simulink model "DhwStationPId3d4"  (R2017a)
settings: Solver=FixedStepAuto  StartTime=-100  StopTime=100  FixedStep=dt  RelTol=1e-3
values from neighbouring files (symbols this model uses):
  A_0 = [ 0.7687, 0,      0,      0.1258, 0,      0,      12.31;          0.1054, 0.7687, 0,      0,      0.1258, 0,      12.31;          0,      0.1054, 0.7687, 0,      0,      0.1258, 12.31;          0.1161, 0,      0,      0.7867, 0.0972, 0,      0.7009;          0,      0.1161, 0,      0,      0.7867, 0.0972, 0.7009;          0,      0,      0.1161, 0,      0,      0.7867, 0.7009;          0,      0,  ...(+44 chars)    [LoadTruncatedSystemMatrices.m]
  A_1 = [	0,  0,  0,  0,  0,  0,  1.054;          0,  0,  0,  0,  0,  0,  0;          0,  0,  0,  0,  0,  0,  0;          0,  0,  0,  0,  0,  0,  0;          0,  0,  0,  0,  0,  0,  0;          0,  0,  0,  0,  0,  0,  0;          0,  0,  0,  0,  0,  0,  0]    [LoadTruncatedSystemMatrices.m]
  A_3 = 1e-3*[    -0.0597,0,      0,      0.0597,     0,  0,      0;                  0,      -0.0597,0,      0,      0.0597, 0,      0;                  0,      0,      -0.0597,0,      0,      0.0597, 0;                  0.0551, 0,      0 ,     -972.4, 972.4,  0,      0;                  0,      0.0551, 0,      0,      -972.4, 972.4,  0;                  0,      0, 0.0551,      0,      0,      -972.4, 0; ...(+68 chars)    [LoadTruncatedSystemMatrices.m]
  A_4 = [ -1.127, 0     , 0,      0.0731, 0,      0,          0;          1.054,  -1.127, 0,      0,      0.0731, 0,          0;          0,      1.054,  -1.127, 0,      0,      0.0731,     0;          0.0675, 0,      0,      -0.0675,0,      0,          0;          0,      0.0675, 0,      0,      -0.0675,0,          0;          0,      0,      0.0675, 0,      0,      -0.0675,    0;          0,      0,     ...(+40 chars)    [LoadTruncatedSystemMatrices.m]
  B_0 = [	0,	0,	0,	0,	0,	0, 0.1]'    [LoadTruncatedSystemMatrices.m]
  C = [0, 0, 0, 1, 0,  0,  0]    [LoadTruncatedSystemMatrices.m]
  d_0 = [70, 	10, 0.1, 0.1]    [LoadTruncatedSystemMatrices.m]
  dt = 0.1    [LoadTruncatedSystemMatrices.m]
  G_1 = [0.1054,	0,	0,	0,	0,	0,	0]'    [LoadTruncatedSystemMatrices.m]
  G_2 = [0, 0, 0,	0, 0, 0.0972, 0]'    [LoadTruncatedSystemMatrices.m]
  G_23 = [ 0,	0,	0,	0,	0, 0.9724,	0]'    [LoadTruncatedSystemMatrices.m]
  G_3 = [ -.0006,	-.0006,	-.0006,	-12.05,	-12.05,	-12.05, 0]'    [LoadTruncatedSystemMatrices.m]
  PId3d4_Ki = 0.000139128218356    [OptimizationReults_GainScheduledPId3d4.mat]    (also in OptimizeGainScheduledPId3d4.m = double(Ki))
  PId3d4_Kid3 = 0.000268812937216    [OptimizationReults_GainScheduledPId3d4.mat]    (also in OptimizeGainScheduledPId3d4.m = double(Kid3))
  PId3d4_Kid3d4 = -0.000522259839167    [OptimizationReults_GainScheduledPId3d4.mat]    (also in OptimizeGainScheduledPId3d4.m = double(Kid3d4))
  PId3d4_Kid4 = 0.000317478765518    [OptimizationReults_GainScheduledPId3d4.mat]    (also in OptimizeGainScheduledPId3d4.m = double(Kid4))
  PId3d4_Kp = 0.0070026798963    [OptimizationReults_GainScheduledPId3d4.mat]    (also in OptimizeGainScheduledPId3d4.m = double(Kp))
  PId3d4_Kpd3 = -0.00260700779742    [OptimizationReults_GainScheduledPId3d4.mat]    (also in OptimizeGainScheduledPId3d4.m = double(Kpd3))
  PId3d4_Kpd3d4 = -0.0177923584549    [OptimizationReults_GainScheduledPId3d4.mat]    (also in OptimizeGainScheduledPId3d4.m = double(Kpd3d4))
  PId3d4_Kpd4 = -0.00285749425693    [OptimizationReults_GainScheduledPId3d4.mat]    (also in OptimizeGainScheduledPId3d4.m = double(Kpd4))
  u_0 = 0.1    [LoadTruncatedSystemMatrices.m]
  x_0 = [ 57.5979, 45.1957, 32.7936,	47.2064, 34.8043, 22.4021, 0.1]'    [LoadTruncatedSystemMatrices.m]
  y_0 = C*x_0    [LoadTruncatedSystemMatrices.m]
settings Model: Creator=tgrunert  LastModifiedBy=tgrunert
settings OptimizationCC: DefaultParameterBehavior=Inlined

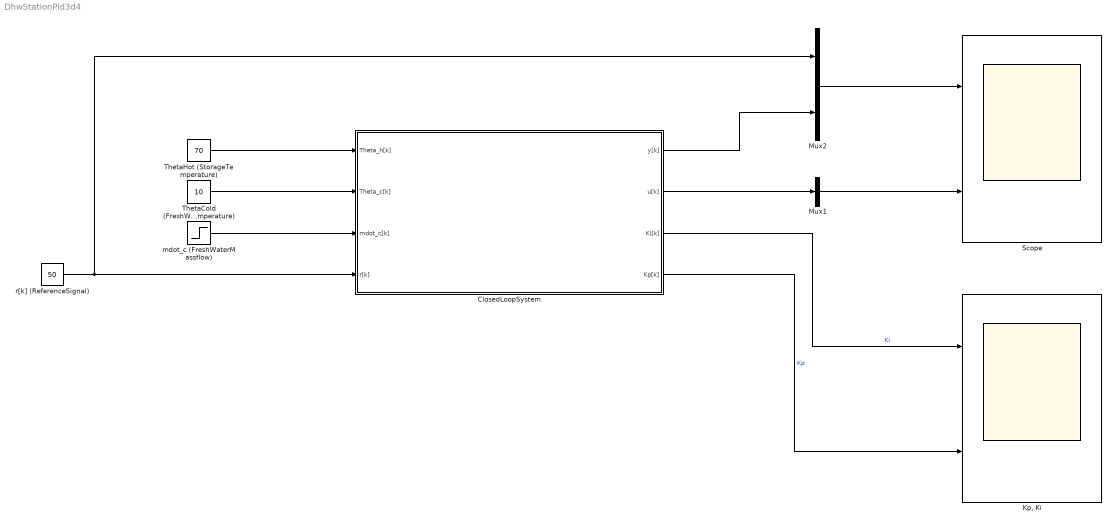
== system DhwStationPId3d4 ==
  ClosedLoopSystem : Subsystem
  "Kp, Ki" : Scope  NumInputPorts=2
  Mux1 : Mux  Inputs=1
  Mux2 : Mux  Inputs=2
  Scope : Scope  NumInputPorts=2
  ThetaCold (FreshWaterTemperature) : Constant  Value=10
  ThetaHot (StorageTemperature) : Constant  Value=70
  mdot_c (FreshWaterMassflow) : Step  Time=0  Before=0.125  After=0.075  SampleTime=0
  r[k] (ReferenceSignal) : Constant  Value=50
  wires:
  Mux1/1 -> Scope/2
  Mux2/1 -> Scope/1
  r[k] (ReferenceSignal)/1 -> Mux2/1, ClosedLoopSystem/4(r[k])
  ThetaCold (FreshWaterTemperature)/1 -> ClosedLoopSystem/2(Theta_c[k])
  ClosedLoopSystem/1(y[k]) -> Mux2/2
  ClosedLoopSystem/2(u[k]) -> Mux1/1
  ThetaHot (StorageTemperature)/1 -> ClosedLoopSystem/1(Theta_h[k])
  mdot_c (FreshWaterMassflow)/1 -> ClosedLoopSystem/3(mdot_c[k])
  ClosedLoopSystem/3(Ki[k]) -> "Kp, Ki"/1  "Ki"
  ClosedLoopSystem/4(Kp[k]) -> "Kp, Ki"/2  "Kp"

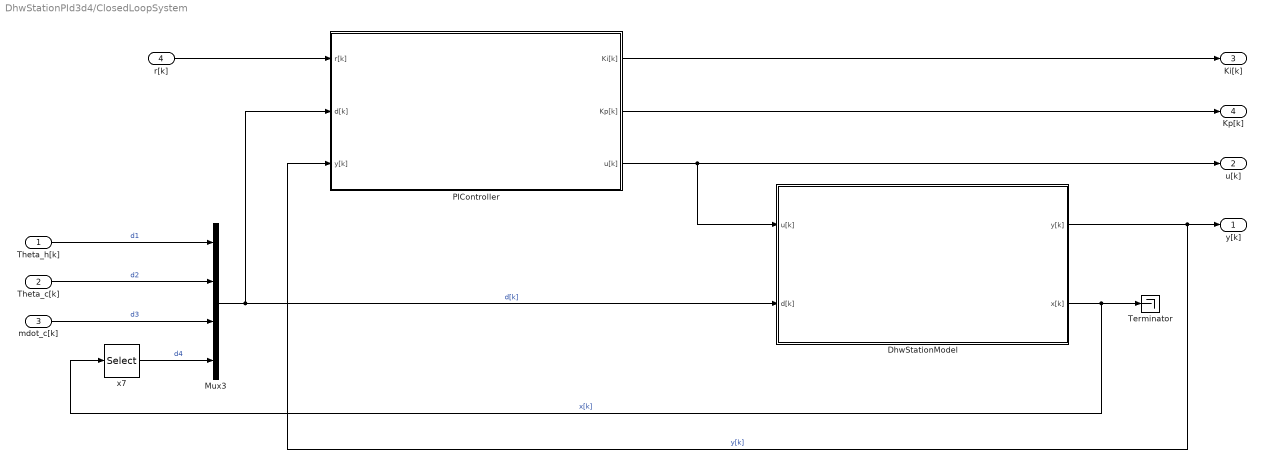
== system DhwStationPId3d4/ClosedLoopSystem ==
  Theta_h[k] : Inport
  Theta_c[k] : Inport  Port=2
  mdot_c[k] : Inport  Port=3
  r[k] : Inport  Port=4
  DhwStationModel : Subsystem  SystemSampleTime=dt
  Mux3 : Mux
  PIController : Subsystem
  Terminator : Terminator
  x7 : Selector  InputPortWidth=7  IndexOptions=Index vector (dialog)  Indices=[7]  OutputSizes=1
  y[k] : Outport
  u[k] : Outport  Port=2
  Ki[k] : Outport  Port=3
  Kp[k] : Outport  Port=4
  wires:
  PIController/3(u[k]) -> u[k]/1, DhwStationModel/1(u[k])
  DhwStationModel/2(x[k]) -> x7/1, Terminator/1  "x[k]"
  Theta_c[k]/1 -> Mux3/2  "d2"
  DhwStationModel/1(y[k]) -> y[k]/1, PIController/3(y[k])  "y[k]"
  Theta_h[k]/1 -> Mux3/1  "d1"
  mdot_c[k]/1 -> Mux3/3  "d3"
  Mux3/1 -> PIController/2(d[k]), DhwStationModel/2(d[k])  "d[k]"
  r[k]/1 -> PIController/1(r[k])
  x7/1 -> Mux3/4  "d4"
  PIController/1(Ki[k]) -> Ki[k]/1
  PIController/2(Kp[k]) -> Kp[k]/1

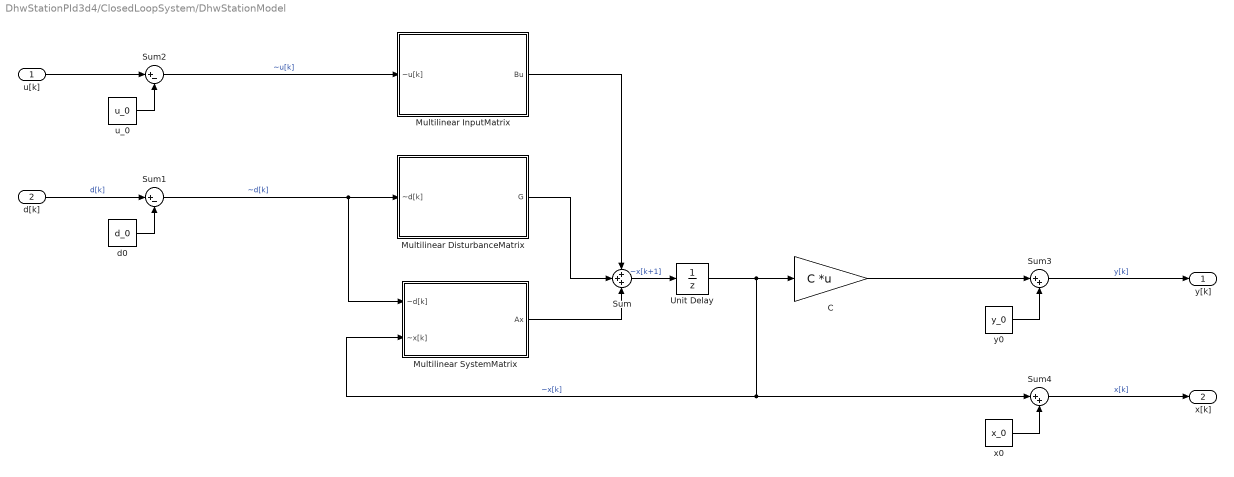
== system DhwStationPId3d4/ClosedLoopSystem/DhwStationModel ==
  u[k] : Inport
  d[k] : Inport  Port=2
  C : Gain  Gain=C  Multiplication=Matrix(K*u) (u vector)
  Multilinear DisturbanceMatrix : Subsystem
  Multilinear InputMatrix : Subsystem
  Multilinear SystemMatrix : Subsystem
  Sum : Sum  Inputs=+++
  Sum1 : Sum  Inputs=|+-
  Sum2 : Sum  Inputs=|+-
  Sum3 : Sum  Inputs=|++
  Sum4 : Sum  Inputs=|++
  Unit Delay : UnitDelay  SampleTime=-1
  d0 : Constant  Value=d_0
  u_0 : Constant  Value=u_0
  "x0 " : Constant  Value=x_0
  y0 : Constant  Value=y_0
  y[k] : Outport  PortDimensions=1
  x[k] : Outport  Port=2
  wires:
  Sum4/1 -> x[k]/1  "x[k]"
  "x0 "/1 -> Sum4/2
  y0/1 -> Sum3/2
  Sum3/1 -> y[k]/1  "y[k]"
  d0/1 -> Sum1/2
  d[k]/1 -> Sum1/1  "d[k]"
  C/1 -> Sum3/1
  Multilinear InputMatrix/1(Bu) -> Sum/1
  Multilinear SystemMatrix/1(Ax) -> Sum/3
  Unit Delay/1 -> Multilinear SystemMatrix/2(~x[k]), Sum4/1, C/1  "~x[k]"
  Sum/1 -> Unit Delay/1  "~x[k+1]"
  u[k]/1 -> Sum2/1
  u_0/1 -> Sum2/2
  Sum2/1 -> Multilinear InputMatrix/1(~u[k])  "~u[k]"
  Multilinear DisturbanceMatrix/1(G) -> Sum/2
  Sum1/1 -> Multilinear SystemMatrix/1(~d[k]), Multilinear DisturbanceMatrix/1(~d[k])  "~d[k]"

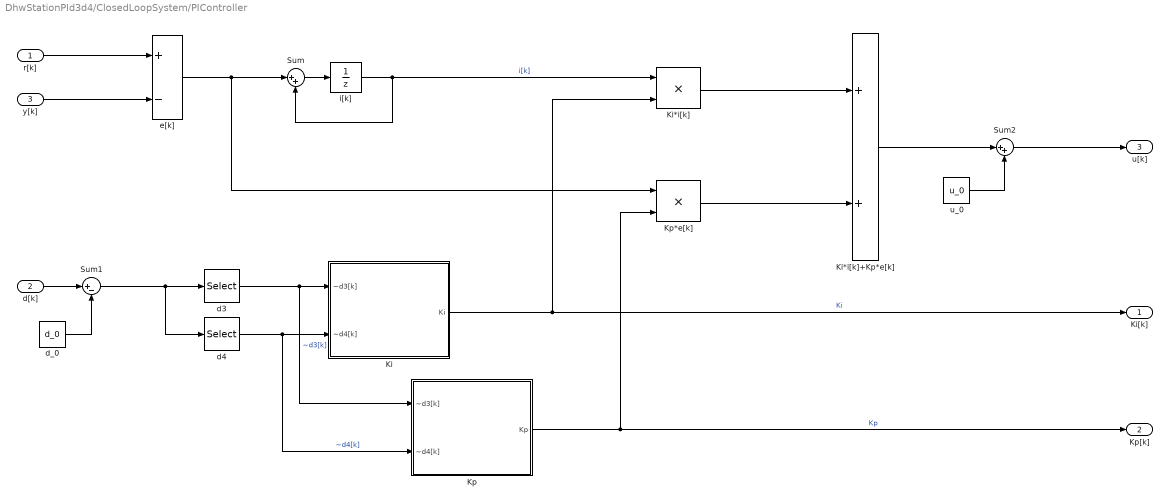
== system DhwStationPId3d4/ClosedLoopSystem/PIController ==
  r[k] : Inport
  d[k] : Inport  Port=2
  y[k] : Inport  Port=3
  Ki : Subsystem
  Ki*i[k] : Product
  Ki*i[k]+Kp*e[k] : Sum
  Kp : Subsystem
  Kp*e[k] : Product
  Sum : Sum  Inputs=|++
  Sum1 : Sum  Inputs=|+-
  Sum2 : Sum  Inputs=|++
  d3 : Selector  InputPortWidth=4  IndexOptions=Index vector (dialog)  Indices=[3]  OutputSizes=1
  d4 : Selector  InputPortWidth=4  IndexOptions=Index vector (dialog)  Indices=[4]  OutputSizes=1
  d_0 : Constant  Value=d_0
  e[k] : Sum  Inputs=+-
  i[k] : UnitDelay  SampleTime=-1
  u_0 : Constant  Value=u_0
  Ki[k] : Outport
  Kp[k] : Outport  Port=2
  u[k] : Outport  Port=3
  wires:
  r[k]/1 -> e[k]/1
  y[k]/1 -> e[k]/2
  e[k]/1 -> Kp*e[k]/1, Sum/1
  Sum/1 -> i[k]/1
  i[k]/1 -> Sum/2, Ki*i[k]/1  "i[k]"
  Sum1/1 -> d3/1, d4/1
  d[k]/1 -> Sum1/1
  d_0/1 -> Sum1/2
  d3/1 -> Ki/1(~d3[k]), Kp/1(~d3[k])  "~d3[k]"
  d4/1 -> Ki/2(~d4[k]), Kp/2(~d4[k])  "~d4[k]"
  Ki/1(Ki) -> Ki*i[k]/2, Ki[k]/1  "Ki"
  Kp/1(Kp) -> Kp[k]/1, Kp*e[k]/2  "Kp"
  Ki*i[k]/1 -> Ki*i[k]+Kp*e[k]/1
  Kp*e[k]/1 -> Ki*i[k]+Kp*e[k]/2
  Ki*i[k]+Kp*e[k]/1 -> Sum2/1
  Sum2/1 -> u[k]/1
  u_0/1 -> Sum2/2

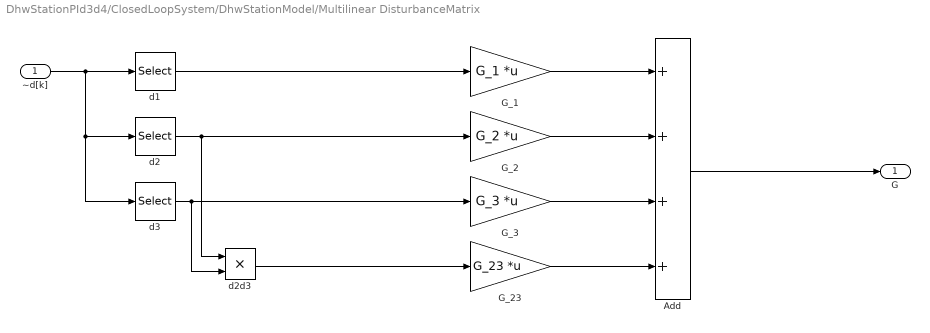
== system DhwStationPId3d4/ClosedLoopSystem/DhwStationModel/Multilinear DisturbanceMatrix ==
  ~d[k] : Inport
  Add : Sum  Inputs=++++
  G_1 : Gain  Gain=G_1  Multiplication=Matrix(K*u)
  G_2 : Gain  Gain=G_2  Multiplication=Matrix(K*u)
  G_23 : Gain  Gain=G_23  Multiplication=Matrix(K*u)
  G_3 : Gain  Gain=G_3  Multiplication=Matrix(K*u)
  d1 : Selector  InputPortWidth=4  IndexOptions=Index vector (dialog)  Indices=[1]  OutputSizes=1
  d2 : Selector  InputPortWidth=4  IndexOptions=Index vector (dialog)  Indices=[2]  OutputSizes=1
  d2d3 : Product
  d3 : Selector  InputPortWidth=4  IndexOptions=Index vector (dialog)  Indices=[3]  OutputSizes=1
  G : Outport
  wires:
  G_1/1 -> Add/1
  ~d[k]/1 -> d2/1, d3/1, d1/1
  d1/1 -> G_1/1
  d2/1 -> d2d3/1, G_2/1
  d3/1 -> d2d3/2, G_3/1
  G_2/1 -> Add/2
  G_3/1 -> Add/3
  d2d3/1 -> G_23/1
  G_23/1 -> Add/4
  Add/1 -> G/1

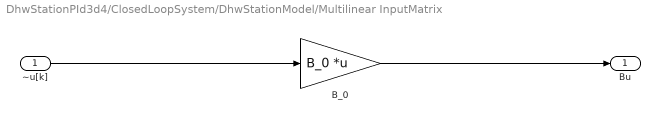
== system DhwStationPId3d4/ClosedLoopSystem/DhwStationModel/Multilinear InputMatrix ==
  ~u[k] : Inport  PortDimensions=1
  B_0 : Gain  Gain=B_0  Multiplication=Matrix(K*u)
  Bu : Outport
  wires:
  ~u[k]/1 -> B_0/1
  B_0/1 -> Bu/1

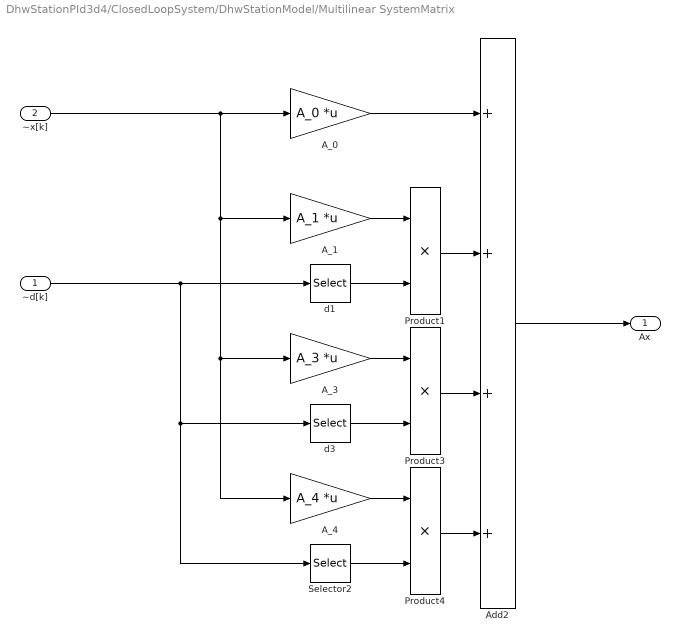
== system DhwStationPId3d4/ClosedLoopSystem/DhwStationModel/Multilinear SystemMatrix ==
  ~d[k] : Inport
  ~x[k] : Inport  Port=2
  A_0 : Gain  Gain=A_0  Multiplication=Matrix(K*u) (u vector)
  A_1 : Gain  Gain=A_1  Multiplication=Matrix(K*u) (u vector)
  A_3 : Gain  Gain=A_3  Multiplication=Matrix(K*u) (u vector)
  A_4 : Gain  Gain=A_4  Multiplication=Matrix(K*u) (u vector)
  Add2 : Sum  Inputs=++++
  Product1 : Product
  Product3 : Product
  Product4 : Product
  Selector2 : Selector  InputPortWidth=4  IndexOptions=Index vector (dialog)  Indices=[4]  OutputSizes=1
  d1 : Selector  InputPortWidth=4  IndexOptions=Index vector (dialog)  Indices=[1]  OutputSizes=1
  d3 : Selector  InputPortWidth=4  IndexOptions=Index vector (dialog)  Indices=[3]  OutputSizes=1
  Ax : Outport
  wires:
  Selector2/1 -> Product4/2
  A_4/1 -> Product4/1
  Product4/1 -> Add2/4
  Product3/1 -> Add2/3
  Product1/1 -> Add2/2
  A_1/1 -> Product1/1
  Add2/1 -> Ax/1
  d3/1 -> Product3/2
  A_0/1 -> Add2/1
  ~x[k]/1 -> A_0/1, A_1/1, A_3/1, A_4/1
  d1/1 -> Product1/2
  A_3/1 -> Product3/1
  ~d[k]/1 -> d1/1, Selector2/1, d3/1

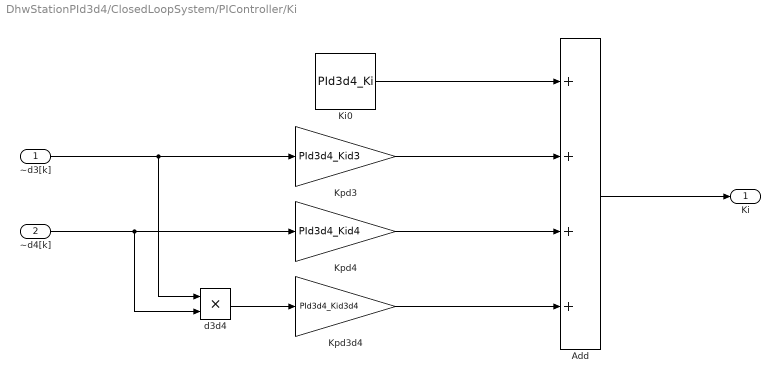
== system DhwStationPId3d4/ClosedLoopSystem/PIController/Ki ==
  ~d3[k] : Inport
  ~d4[k] : Inport  Port=2
  Add : Sum  Inputs=++++
  Ki0 : Constant  Value=PId3d4_Ki
  Kpd3 : Gain  Gain=PId3d4_Kid3
  Kpd3d4 : Gain  Gain=PId3d4_Kid3d4
  Kpd4 : Gain  Gain=PId3d4_Kid4
  d3d4 : Product
  Ki : Outport
  wires:
  Add/1 -> Ki/1
  Kpd3/1 -> Add/2
  Ki0/1 -> Add/1
  d3d4/1 -> Kpd3d4/1
  Kpd3d4/1 -> Add/4
  Kpd4/1 -> Add/3
  ~d3[k]/1 -> Kpd3/1, d3d4/1
  ~d4[k]/1 -> Kpd4/1, d3d4/2

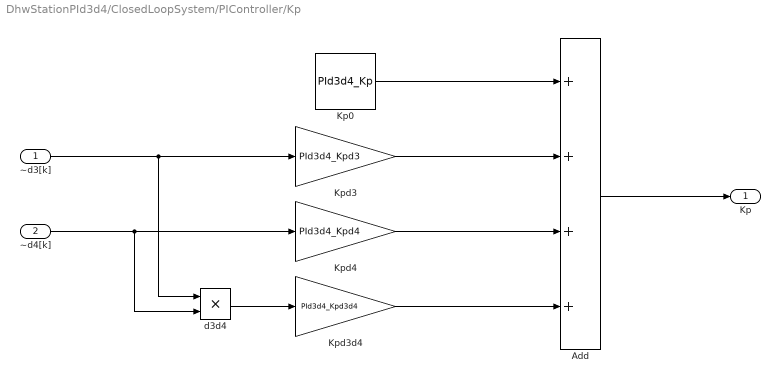
== system DhwStationPId3d4/ClosedLoopSystem/PIController/Kp ==
  ~d3[k] : Inport
  ~d4[k] : Inport  Port=2
  Add : Sum  Inputs=++++
  Kp0 : Constant  Value=PId3d4_Kp
  Kpd3 : Gain  Gain=PId3d4_Kpd3
  Kpd3d4 : Gain  Gain=PId3d4_Kpd3d4
  Kpd4 : Gain  Gain=PId3d4_Kpd4
  d3d4 : Product
  Kp : Outport
  wires:
  ~d4[k]/1 -> d3d4/2, Kpd4/1
  ~d3[k]/1 -> d3d4/1, Kpd3/1
  Kpd4/1 -> Add/3
  Kpd3d4/1 -> Add/4
  d3d4/1 -> Kpd3d4/1
  Kp0/1 -> Add/1
  Kpd3/1 -> Add/2
  Add/1 -> Kp/1
